simulink model "Week3_problem_3"  (R2020b)
settings: Solver=VariableStepAuto  StartTime=0.0  StopTime=10.0  RelTol=1e-3
PreLoadFcn:
  |  m=75
  | v0=44
  | R=1.25
  | g=9.81
undefined symbols (not defined in the file): I
settings Model: Creator=sai  LastModifiedBy=sai

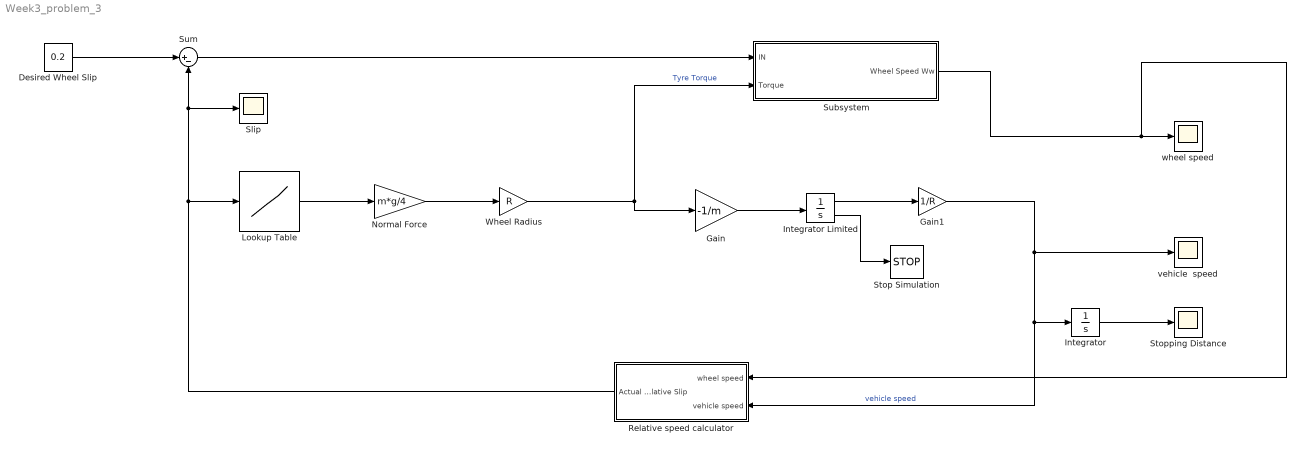
== system Week3_problem_3 ==
  Desired Wheel Slip : Constant  Value=0.2
  Gain : Gain  Gain=-1/m
  Gain1 : Gain  Gain=1/R
  Integrator : Integrator
  Integrator Limited : Integrator  InitialCondition=v0/R  LimitOutput=on  UpperSaturationLimit=1000  LowerSaturationLimit=0  ShowSaturationPort=on
  Lookup Table : Lookup_n-D  NumberOfTableDimensions=1  BreakpointsForDimension1=[0,0.05,0.1,0.15,0.2,0.25,0.3,0.35,0.4,0.45,0.5,0.55,0.6,0.65,0.7,0.75,0.8,0.85,0.9,0.95,1]  Table=[0,0.4,0.8,0.97,1,0.98,0.96,0.94,0.92,0.9,0.88,0.855,0.83,0.81,0.79,0.77,0.75,0.73,0.72,0.71,0.7]  InternalRulePriority=Speed  RndMeth=Simplest  InputSameDT=on
  "Normal Force " : Gain  Gain=m*g/4
  Relative speed calculator : Subsystem
  Slip : Scope
  Stop Simulation : Stop
  Stopping Distance : Scope
  Subsystem : Subsystem
  Sum : Sum  Inputs=|+-
  Wheel Radius : Gain  Gain=R
  vehicle  speed : Scope
  wheel speed : Scope
  wires:
  Sum/1 -> Subsystem/1(IN)
  Gain/1 -> Integrator Limited/1
  Integrator Limited/2 -> Stop Simulation/1
  Relative speed calculator/1(Actual Relative Slip) -> Lookup Table/1, Slip/1, Sum/2
  Wheel Radius/1 -> Gain/1, Subsystem/2(" Torque")  "Tyre Torque"
  Desired Wheel Slip/1 -> Sum/1
  Lookup Table/1 -> "Normal Force "/1
  Integrator/1 -> Stopping Distance/1
  "Normal Force "/1 -> Wheel Radius/1
  Gain1/1 -> vehicle  speed/1, Relative speed calculator/2(vehicle speed), Integrator/1  "vehicle speed"
  Integrator Limited/1 -> Gain1/1
  Subsystem/1(Wheel Speed Ww) -> wheel speed/1, Relative speed calculator/1(wheel speed)

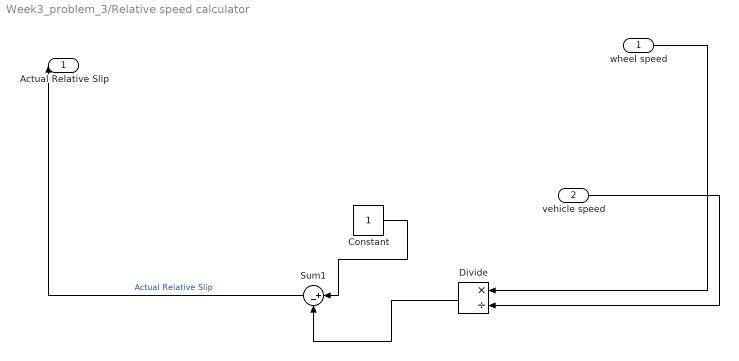
== system Week3_problem_3/Relative speed calculator ==
  wheel speed : Inport
  vehicle speed : Inport  Port=2
  Constant : Constant
  Divide : Product  Inputs=*/
  Sum1 : Sum  Inputs=|+-
  Actual Relative Slip : Outport
  wires:
  Sum1/1 -> Actual Relative Slip/1  "Actual Relative Slip"
  wheel speed/1 -> Divide/1
  Constant/1 -> Sum1/1
  Divide/1 -> Sum1/2
  vehicle speed/1 -> Divide/2

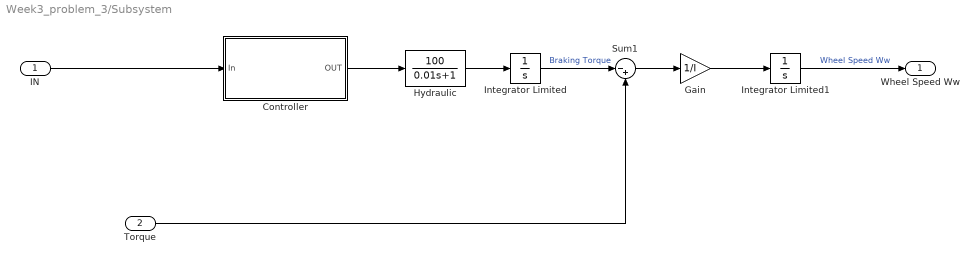
== system Week3_problem_3/Subsystem ==
  IN : Inport
  " Torque" : Inport  Port=2
  Controller : Subsystem
  Gain : Gain  Gain=1/I
  "Hydraulic " : TransferFcn  Numerator=[100]  Denominator=[0.01 1]
  Integrator Limited : Integrator  LimitOutput=on  UpperSaturationLimit=1000  LowerSaturationLimit=0
  Integrator Limited1 : Integrator  InitialCondition=v0/R  LimitOutput=on  UpperSaturationLimit=1000  LowerSaturationLimit=0
  Sum1 : Sum  Inputs=|-+
  Wheel Speed Ww : Outport
  wires:
  Controller/1(OUT) -> "Hydraulic "/1
  " Torque"/1 -> Sum1/2
  "Hydraulic "/1 -> Integrator Limited/1
  Integrator Limited/1 -> Sum1/1  "Braking Torque"
  IN/1 -> Controller/1(In)
  Integrator Limited1/1 -> Wheel Speed Ww/1  "Wheel Speed Ww"
  Sum1/1 -> Gain/1
  Gain/1 -> Integrator Limited1/1

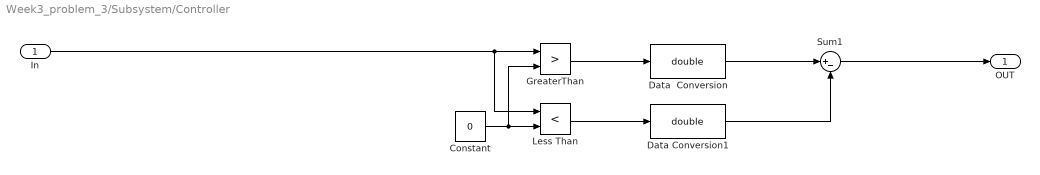
== system Week3_problem_3/Subsystem/Controller ==
  In : Inport
  Constant : Constant  Value=0
  "Data  Conversion " : DataTypeConversion  OutDataTypeStr=double  RndMeth=Zero
  "Data Conversion1 " : DataTypeConversion  OutDataTypeStr=double  RndMeth=Zero
  "GreaterThan " : RelationalOperator  Operator=>  OutDataTypeStr=boolean  RndMeth=Simplest
  "Less Than " : RelationalOperator  Operator=<  OutDataTypeStr=boolean  RndMeth=Simplest
  Sum1 : Sum  Inputs=|+-
  OUT : Outport
  wires:
  "GreaterThan "/1 -> "Data  Conversion "/1
  In/1 -> "Less Than "/1, "GreaterThan "/1
  "Data Conversion1 "/1 -> Sum1/2
  Sum1/1 -> OUT/1
  "Less Than "/1 -> "Data Conversion1 "/1
  "Data  Conversion "/1 -> Sum1/1
  Constant/1 -> "GreaterThan "/2, "Less Than "/2
